simulink model "pid_simulation"  (R2023b)
settings: Solver=FixedStepAuto  StartTime=0.0  StopTime=600  FixedStep=1  RelTol=1e-3
values from neighbouring files (symbols this model uses):
  delay = 10    [pid_values.m]
  dt = 1.0    (= 1)    [pid_values.m]
  initial_value = 19    [pid_values.m]
  k = 12.746    [pid_values.m]
  kd = 0.0122    [pid_values.m]
  ki = 0.0035    [pid_values.m]
  kp = 0.3073    [pid_values.m]
  set_point = 25    [pid_values.m]
  T = 190    [pid_values.m]
settings Model: Creator=dawidexpompa2000  LastModifiedBy=Marci
settings DebuggingCC: UnconnectedInputMsg=warning  UnconnectedOutputMsg=warning  UnconnectedLineMsg=warning
settings ModelReferenceCC: EnableRefExpFcnMdlSchedulingChecks=on
settings RTWCC: DLArmComputeVersion=19.05

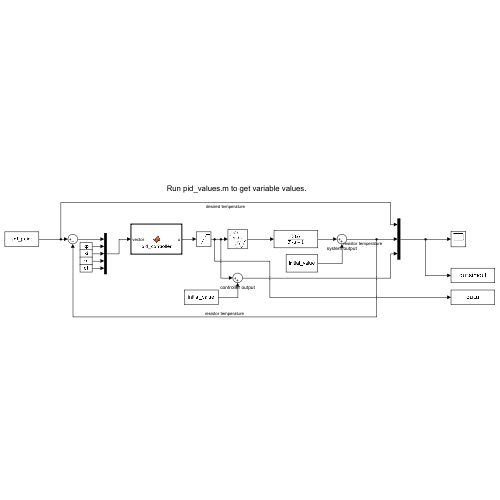
[thumbnail: Simulink's stored preview of the top-level diagram]
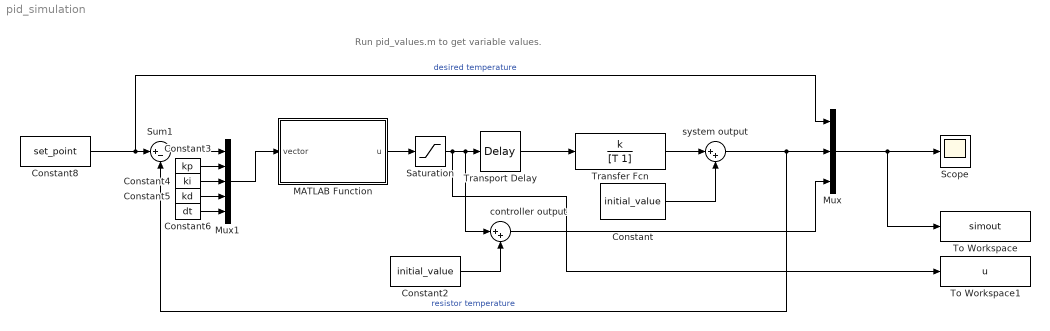
== system pid_simulation ==
  note: Run pid_values.m to get variable values.
  Constant : Constant  Value=initial_value
  Constant2 : Constant  Value=initial_value
  Constant3 : Constant  Value=kp
  Constant4 : Constant  Value=ki
  Constant5 : Constant  Value=kd
  Constant6 : Constant  Value=dt
  Constant8 : Constant  Value=set_point
  MATLAB Function : MATLAB Function  TreatAsAtomicUnit=on
  Mux : Mux  Inputs=3
  Mux1 : Mux  Inputs=5
  Saturation : Saturate  UpperLimit=1  LowerLimit=0
  Scope : Scope
  Sum1 : Sum  Inputs=|+-
  To Workspace : ToWorkspace  VariableName=simout  SaveFormat=Timeseries  SampleTime=-1
  To Workspace1 : ToWorkspace  VariableName=u  SaveFormat=Timeseries  SampleTime=-1
  Transfer Fcn : TransferFcn  Numerator=k  Denominator=[T 1]
  Transport Delay : TransportDelay  DelayTime=delay
  controller output : Sum  Inputs=|++
  system output : Sum  Inputs=|++
  wires:
  Transport Delay/1 -> Transfer Fcn/1
  Transfer Fcn/1 -> system output/1
  Constant/1 -> system output/2
  system output/1 -> Sum1/2, Mux/2  "resistor temperature"
  Mux/1 -> To Workspace/1, Scope/1
  Constant8/1 -> Mux/1, Sum1/1  "desired temperature"
  controller output/1 -> Mux/3
  Constant2/1 -> controller output/2
  Saturation/1 -> To Workspace1/1, controller output/1, Transport Delay/1
  MATLAB Function/1(u) -> Saturation/1
  Mux1/1 -> MATLAB Function/1(vector)
  Sum1/1 -> Mux1/1
  Constant3/1 -> Mux1/2
  Constant4/1 -> Mux1/3
  Constant5/1 -> Mux1/4
  Constant6/1 -> Mux1/5

== matlab function pid_simulation/MATLAB Function ==
  settings: updateMethod=DISCRETE
  data: vector input; u output
function u = pid_controller(vector)
%separate data from passed vector:
e = vector(1);
kp = vector(2);
ki = vector(3);
kd = vector(4);
dt = vector(5);

%static value
persistent previous_error;
if isempty(previous_error)
    previous_error = 0;
end

persistent previous_integral;
if isempty(previous_integral)
    previous_integral = 0;
end

%controller equations:
%proprotional part
P = kp*e;

%integral part
integral = previous_integral + (e+previous_error) ; %numerical integrator without anti-windup
previous_integral = integral;
I = ki*integral*(dt/2);

%derivative part
derivative = (e - previous_error)/dt;
previous_error = e;
D = kd*derivative;


u = P + I + D;
